simulink model "drone_sim"  (R2021a)
settings: Solver=VariableStepAuto  StartTime=0.0  StopTime=5  MaxStep=0.001  RelTol=1e-7  EnableMultiTasking=on
values from neighbouring files (symbols this model uses):
  arm_length = motorY    (= 0.37)    [drone_6.m]
  batteryDistanceFromCOG = -0.1    [drone_6.m]
  batteryMass = 0.5    [drone_6.m]
  batVolt = 3.7*cells    (= 11.1)    [drone_6.m]
  bodyMass = 0.3    [drone_6.m]
  deadCurrent = 0.3    [drone_6.m]
  h1al = 0.15    [drone_6.m]
  h1iuse = 0    [drone_6.m]
  h1kp = 0    [drone_6.m]
  h1td = 1    [drone_6.m]
  h1ti = 1000    [drone_6.m]
  hoverControl = hoverVoltage/batVolt*1024    [drone_6.m]
  hoverVoltage = hoverCurrent * Ra + hoverRPM / Kv    [drone_6.m]
  hval = 0.2    [drone_6.m]
  hviuse = 0    [drone_6.m]
  hvkp = 50    [drone_6.m]
  hvtd = 1    [drone_6.m]
  hvti = 1    [drone_6.m]
  KDrag = 1.5e-9    (= 1.5e-09)    [drone_6.m]
  Km = 60/(Kv * 2 * pi)    (= 0.013641852265)    [drone_6.m]
  Ktrust = 2.7e-5    (= 2.7e-05)    [drone_6.m]
  minimumMotorVolt = 1.0    (= 1)    [drone_6.m]
  motorMass = 0.102    [drone_6.m]
  N = N + 1    (= 1)    [findp_discrete.m]    (also in findpd_discrete.m = N0; findpi_discrete.m; findpid_discrete.m)
  paal = 0.2    [drone_6.m]
  pakp = 0    [drone_6.m]
  patd = 1    [drone_6.m]
  pati = 100    [drone_6.m]
  pitch_act_lim = 500    [drone_6.m]
  propellerMass = propellerMassRaw + 3*motorInertia/propellerRadius^2    (= 0.019780754243)    [drone_6.m]
  pushOn = 1    [drone_6.m]
  pv_iuse = 0    [drone_6.m]
  pval = 0.4    [drone_6.m]
  pvkp = 0    [drone_6.m]
  pvtd = 1    [drone_6.m]
  pvti = 1    [drone_6.m]
  Ra = 0.083    [drone_6.m]
  raal = 0.25    [drone_6.m]
  rakp = 0    [drone_6.m]
  ral = 0.5    [drone_6.m]
  ratd = 1    [drone_6.m]
  rati = 100    [drone_6.m]
  rkp = 0    [drone_6.m]
  roll_act_lim = 500    [drone_6.m]
  roll_limit = 10    [drone_6.m]
  rtd = 1    [drone_6.m]
  rti = 1    [drone_6.m]
  trust_lim = 1000*0.95    (= 950)    [drone_6.m]
  yaw_act_lim = 500    [drone_6.m]
  yaw_rate_limit = 90    [drone_6.m]
  yawval = 0.3    [drone_6.m]
  yawvkp = 0    [drone_6.m]
  yawvtd = 0    [drone_6.m]
  yawvti = 1    [drone_6.m]
  yawvtiUse = 0    [drone_6.m]
undefined symbols (not defined in the file or in its folder): X, Y, Z
libraries: sm_lib x56, nesl_utility x25, sharedtransform x1
(part 1 of 3)
settings Model: OrderedModelArguments=off  Creator=chr  LastModifiedBy=chr
settings SolverCC: AlgebraicLoopSolver=TrustRegion
settings DataIOCC: LimitDataPoints=on  SaveFormat=Array  ReturnWorkspaceOutputs=off
settings OptimizationCC: LifeSpan=inf
settings DebuggingCC: SFUnexpectedBacktrackingDiag=warning  SFNoUnconditionalDefaultTransitionDiag=warning  SFExecutionAtInitializationDiag=none  SFMachineParentedDataDiag=warning  ArithmeticOperatorsInVariantConditions=warning
settings HardwareCC: ProdBitPerPointer=32  ProdBitPerSizeT=32  ProdBitPerPtrDiffT=32  ProdLargestAtomicFloat=None  ProdIntDivRoundTo=Undefined  ProdEndianess=Unspecified  ProdWordSize=32  ProdHWDeviceType=32-bit Generic
settings ModelReferenceCC: PropagateSignalLabelsOutOfModel=off
settings SFSimCC: SimUseLocalCustomCode=off  CustomCodeUndefinedFunction=UseInterfaceOnly
settings RTWCC: RTWUseLocalCustomCode=off
settings CodeAppCC: StateflowObjectComments=on
settings GRTTargetCC: TargetLangStandard=C89/C90 (ANSI)
settings ConfigComp: CovMetricSettings=dw  CovSaveCumulativeToWorkspaceVar=on  CovSaveSingleToWorkspaceVar=on  CovExternalEMLEnable=off
settings SimscapeCC: SimscapeNormalizeSystem=off  SimscapeLogType=all  SimscapeLogDataHistory=10000
settings ConfigurationSet: Description=SimMechanics 2G
settings ExplorerConfigSet: InternalSimMechanicsExplorerSettings="<ExplorerConfiguration><canonicalview>default</canonicalview><AnimationSetting><BasePlaybackSpeed>1.0</BasePlaybackSpeed><PlaybackSpeedFactor>1.0</PlaybackSpeedFactor></AnimationSetting><TilePanel><TileInfo><Tiles Columns=\"1\" Count=\"1\" Rows=\"1\"><Column Weight=\"1\"/><Row Weight=\"1\"/><Tile Height=\"1\" Width=\"1\" X=\"0\" Y=\"0\"/></Tiles></TileInfo><SceneInfo><SceneViewer><BGColor><R>0.800000011920928955</R><G>0.800000011920928955</G><B>0.800000011920928955</B></BGColor><Camera><DoPerspective>off</DoPerspective><Position><X>-3434.85384488270984</X><Y>-3.87132408808614903</Y><Z>0.619625050913271247</Z></Position><Center><X>-0.134324382199702441</X><Y>-3.87132408808614903</Y><Z>0.619625050913271247</Z></Center><Up><X>0</X><Y>0</Y><Z>1</Z></Up><ViewLimDist>1</ViewLimDist><YLim>2.62838632598170996</YLim><XLim>4.25180140967629594</XLim></Camera></SceneViewer></SceneInfo></TilePanel><MechEditorPanel><Cameras/><GfxPanelCameraMap/><VideoCreator><PlaybackSpeedRatio>1.0</PlaybackSpeedRatio><FrameRate>30</FrameRate><VideoFormat>Motion JPEG AVI</VideoFormat><FrameSize>auto</FrameSize></VideoCreator></MechEditorPanel></ExplorerConfiguration>"

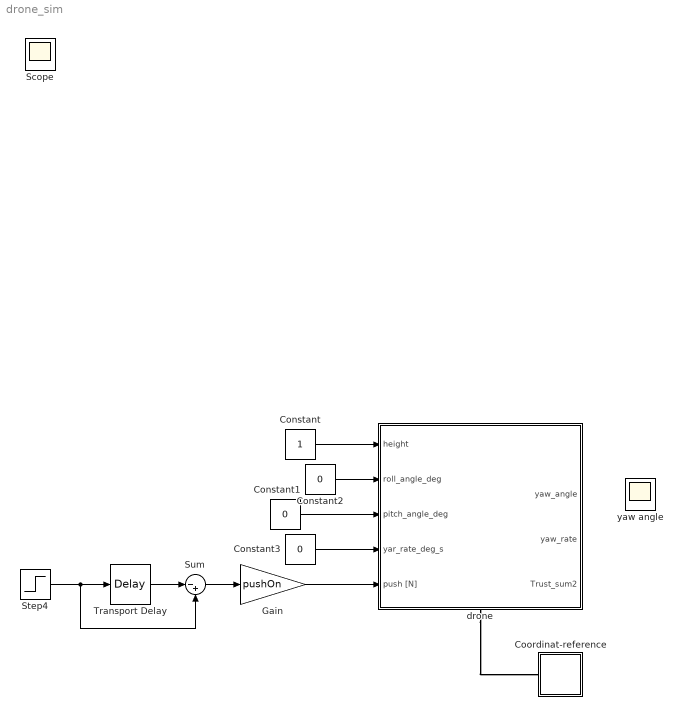
== system drone_sim ==
  Constant : Constant
  Constant1 : Constant  Value=0
  Constant2 : Constant  Value=0
  Constant3 : Constant  Value=0
  Coordinat-reference : Subsystem
  Gain : Gain  Gain=pushOn
  Step4 : Step  Time=2  After=0.2  SampleTime=0
  Sum : Sum  Inputs=|-+
  Transport Delay : TransportDelay  DelayTime=0.2  BufferSize=8196  TransDelayFeedthrough=on
  drone : Subsystem
      settings: PortSchema="{\"entries\":[{\"content\":{\"sides\":[{\"content\":{\"connectorIds\":[\"In1\",\"In2\",\"In3\",\"In4\",\"In5\"]},\"type\":\"ConnectorPlacement.EquallySpacedRectSide\",\"uuid\":\"5594123d-be73-484a-b338-9fd4bc13ca6f\"},{\"content\":{\"connectorIds\":[\"RConn1\",\"Out1\",\"Out2\",\"Out3\"],\"side\":\"RIGHT\"},\"type\":\"ConnectorPlacement.EquallySpacedRectSide\",\"uuid\":\"b12affea-941f-4227-8ac4-f2e96d545e11\"},{\"content\":{\"connectorIds\":[],\"side\":\"TOP\"},\"type\":\"ConnectorPlacement.EquallySpacedRectSide\",\"uuid\":\"44fddaec-2c63-4c5e-8ac9-7d0bb430db34\"},{\"content\":{\"connectorIds\":[\"RConn2\"],\"side\":\"BOTTOM\"},\"type\":\"ConnectorPlacement.EquallySpacedRectSide\",\"uuid\":\"66092044-52c6-48c0-92d2-28ab2c6276b4\"}]},\"type\":\"ConnectorPlacement.EquallySpacedConnector\",\"uuid\":\"500ef50b-769a-4549-99d8-2c1464490163\"}],\"packageUris\":[\"http://schema.mathworks.com/mf0/Connector/R2020b\"],\"version\":\"1.0\"}"
  yaw angle : Scope
  Scope : Scope
  wires:
  Constant/1 -> drone/1(height)
  Step4/1 -> Sum/2, Transport Delay/1
  Transport Delay/1 -> Sum/1
  Sum/1 -> Gain/1
  Constant1/1 -> drone/3(pitch_angle_deg)
  Constant3/1 -> drone/4(yar_rate_deg_s)
  Constant2/1 -> drone/2(roll_angle_deg)
  Gain/1 -> drone/5(push [N])
  connections:
  drone/RConn2 -- Coordinat-reference/RConn1

== system drone_sim/Coordinat-reference ==
  Mechanism Configuration : sm_lib/Utilities/Mechanism Configuration  UniformGravity=Constant  GravityVector=[0 0 -9.82]  GravityVectorUnits=m/s^2  GravityUnits=m/s^2  LinearizationDelta=0.001  JointModeTransitionNonlinearIterations=2
  Solver Configuration : nesl_utility/Solver Configuration  PhysicalDomain=network_engine_domain  SubClassName=solver  LeftPortType=input  RightPortType=generic  Tones=[]  Harmonics=[]  SimulateNoise=off  Profile=off  UseLocalSampling=off  EnableSwitchedLinearOptims=on  FrequencyDomain=off  UseCCode=off  RelTol=0.001  AbsTol=1e-06  MinStep=1e-09  ToWorkspace=off  RevertToSquareIcSolve=off  NumHomotopyIterations=100  PhasorMode=off  PhasorModeNumHarmonics=1  DoDC=off  ResidualTolerance=1e-09  UseLocalSolver=off  LocalSolverChoice=NE_BACKWARD_EULER_ADVANCER  LocalSolverSampleTime=0.001  DoFixedCost=off  MaxNonlinIter=3  MaxModeIter=2  ComputeImpulses=off  ImpulseIterations=2  LinearAlgebra=Sparse  EquationFormulation=NE_TIME_EF  DelaysMemoryBudget=1024  AutomaticFiltering=on  FilteringTimeConstant=0.001  PartitionStorageMethod=AS_NEEDED  PartitionMemoryBudget=1024  PartitionMethod=FAST
      settings: SourceProductBaseCode=PW,SS
  World Frame : sm_lib/Frames and Transforms/World Frame
  ground : sm_lib/Body Elements/Brick Solid  GraphicAmbientColor=[0.15 0.15 0.15 1.0]  BasedOnType=Mass  BrickDimensions=[1 1 0.01]  BrickDimensionUnits=m  CenterOfMass=[0 0 0]  CenterOfMassUnits=m  GraphicDiffuseColor=[0.2 0.5 0.2]  Density=1000  DensityUnits=kg/(m^3)  DoExposeReferenceFrame=on  GraphicEmissiveColor=[0.0 0.0 0.0 1.0]  ExportEntireGeometry=off  SerializedFrames=<Frames/>  MarkerShape=Sphere  MarkerSize=10  GraphicType=FromGeometry  InertiaType=CalculateFromGeometry  Mass=1  MassUnits=kg  MomentsOfInertia=[1 1 1]  MomentsOfInertiaUnits=kg*m^2  GraphicOpacity=1.0  ProductsOfInertia=[0 0 0]  ProductsOfInertiaUnits=kg*m^2  GraphicShininess=75  GraphicSpecularColor=[0.5 0.5 0.5 1.0]  GraphicVisPropType=SimpleVisualProperties
  GND : PMIOPort  Side=Right
  connections:
  Solver Configuration/RConn1 -- GND/RConn1 -- ground/RConn1 -- World Frame/RConn1 -- Mechanism Configuration/RConn1

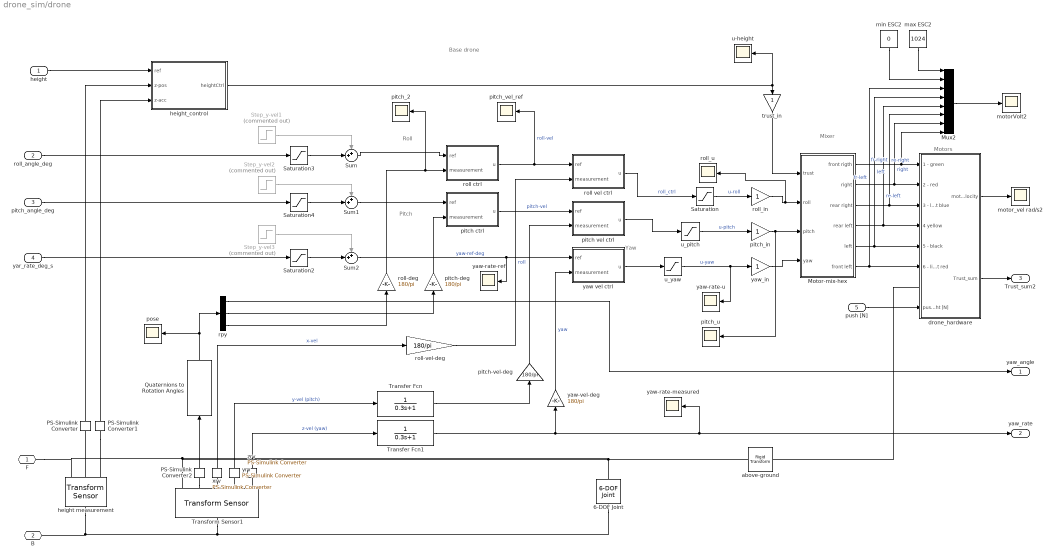
== system drone_sim/drone ==
  note: Base drone
  note: Yaw
  note: Pitch
  note: Roll
  note: Motors
  note: Mixer
  height : Inport
  roll_angle_deg : Inport  Port=2
  pitch_angle_deg : Inport  Port=3
  yar_rate_deg_s : Inport  Port=4
  push [N] : Inport  Port=5
  6-DOF Joint : sm_lib/Joints/6-DOF Joint  JointMode=Normal  SenseConstraintForce=off  SenseConstraintForceX=off  SenseConstraintForceY=off  SenseConstraintForceZ=off  SenseConstraintTorque=off  SenseConstraintTorqueX=off  SenseConstraintTorqueY=off  SenseConstraintTorqueZ=off  SenseTotalForce=off  SenseTotalForceX=off  SenseTotalForceY=off  SenseTotalForceZ=off  SenseTotalTorque=off  SenseTotalTorqueX=off  SenseTotalTorqueY=off  SenseTotalTorqueZ=off  CompositeWrenchDir=FollowerOnBase  CompositeWrenchFrame=BaseFrame  PxEquilibriumPosition=0  PxEquilibriumPositionUnits=m  PxSpringStiffness=0  PxSpringStiffnessUnits=N/m  PxDampingCoefficient=0  PxDampingCoefficientUnits=N/(m/s)  PxTorqueActuationMode=NoTorque  PxMotionActuationMode=ComputedMotion  PxSensePosition=off  PxSenseVelocity=off  PxSenseAcceleration=off  PxSenseTorqueForce=off  PxSenseLowerLimitTorqueForce=off  PxSenseUpperLimitTorqueForce=off  PxLowerLimitSpecify=off  PxLowerLimitBound=-1  PxLowerLimitBoundUnits=m  PxLowerLimitStiffness=1e6  PxLowerLimitStiffnessUnits=N/m  PxLowerLimitDamping=1e3  PxLowerLimitDampingUnits=N/(m/s)  PxLowerLimitTransitionRegionWidth=1e-4  PxLowerLimitTransitionRegionWidthUnits=m  PxUpperLimitSpecify=off  PxUpperLimitBound=1  PxUpperLimitBoundUnits=m  PxUpperLimitStiffness=1e6  PxUpperLimitStiffnessUnits=N/m  PxUpperLimitDamping=1e3  PxUpperLimitDampingUnits=N/(m/s)  PxUpperLimitTransitionRegionWidth=1e-4  PxUpperLimitTransitionRegionWidthUnits=m  PxPositionTargetSpecify=off  PxPositionTargetPriority=High  PxPositionTargetValue=0  PxPositionTargetValueUnits=m  PxVelocityTargetSpecify=off  PxVelocityTargetPriority=High  PxVelocityTargetValue=0  PxVelocityTargetValueUnits=m/s  PyEquilibriumPosition=0  PyEquilibriumPositionUnits=m  PySpringStiffness=0  PySpringStiffnessUnits=N/m  PyDampingCoefficient=0  PyDampingCoefficientUnits=N/(m/s)  PyTorqueActuationMode=NoTorque  PyMotionActuationMode=ComputedMotion  PySensePosition=off  PySenseVelocity=off  PySenseAcceleration=off  PySenseTorqueForce=off  PySenseLowerLimitTorqueForce=off  PySenseUpperLimitTorqueForce=off  PyLowerLimitSpecify=off  PyLowerLimitBound=-1  PyLowerLimitBoundUnits=m  PyLowerLimitStiffness=1e6  PyLowerLimitStiffnessUnits=N/m  PyLowerLimitDamping=1e3  PyLowerLimitDampingUnits=N/(m/s)  PyLowerLimitTransitionRegionWidth=1e-4  PyLowerLimitTransitionRegionWidthUnits=m  PyUpperLimitSpecify=off  PyUpperLimitBound=1  PyUpperLimitBoundUnits=m  PyUpperLimitStiffness=1e6  PyUpperLimitStiffnessUnits=N/m  PyUpperLimitDamping=1e3  PyUpperLimitDampingUnits=N/(m/s)  PyUpperLimitTransitionRegionWidth=1e-4  PyUpperLimitTransitionRegionWidthUnits=m  PyPositionTargetSpecify=off  PyPositionTargetPriority=High  PyPositionTargetValue=0  PyPositionTargetValueUnits=m  PyVelocityTargetSpecify=off  PyVelocityTargetPriority=High  PyVelocityTargetValue=0  PyVelocityTargetValueUnits=m/s  PzEquilibriumPosition=0  PzEquilibriumPositionUnits=m  PzSpringStiffness=0  PzSpringStiffnessUnits=N/m  PzDampingCoefficient=0  PzDampingCoefficientUnits=N/(m/s)  PzTorqueActuationMode=NoTorque  PzMotionActuationMode=ComputedMotion  PzSensePosition=off  PzSenseVelocity=off  PzSenseAcceleration=off  PzSenseTorqueForce=off  PzSenseLowerLimitTorqueForce=off  PzSenseUpperLimitTorqueForce=off  PzLowerLimitSpecify=off  PzLowerLimitBound=-1  PzLowerLimitBoundUnits=m  PzLowerLimitStiffness=1e6  PzLowerLimitStiffnessUnits=N/m  PzLowerLimitDamping=1e3  PzLowerLimitDampingUnits=N/(m/s)  PzLowerLimitTransitionRegionWidth=1e-4  PzLowerLimitTransitionRegionWidthUnits=m  PzUpperLimitSpecify=off  PzUpperLimitBound=1  PzUpperLimitBoundUnits=m  PzUpperLimitStiffness=1e6  PzUpperLimitStiffnessUnits=N/m  PzUpperLimitDamping=1e3  PzUpperLimitDampingUnits=N/(m/s)  PzUpperLimitTransitionRegionWidth=1e-4  PzUpperLimitTransitionRegionWidthUnits=m  PzPositionTargetSpecify=off  PzPositionTargetPriority=High  PzPositionTargetValue=0  PzPositionTargetValueUnits=m  PzVelocityTargetSpecify=off  PzVelocityTargetPriority=High  PzVelocityTargetValue=0  PzVelocityTargetValueUnits=m/s  SphDefPosRotationMethod=None  SphDefPosRotationAngleUnits=deg  SphDefPosRotationStandardAxis=+Z  SphDefPosRotationAngle=0.0  SphDefPosRotationArbitraryAxis=[0 0 1]  SphDefPosFollAlignAxisA=+X  SphDefPosBaseAlignAxisA=+Y  SphDefPosFollAlignAxisB=+Y  SphDefPosBaseAlignAxisB=+Z  SphDefPosRotationSequenceAxes=FollowerAxes  SphDefPosRotationSequence=XYX  SphDefPosRotationSequenceAngles=[0 0 0]  SphDefPosRotationSequenceAnglesUnits=deg  SphDefPosRotationMatrix=[1 0 0; 0 1 0; 0 0 1]  SphEqPosRotationMethod=None  SphEqPosRotationAngleUnits=deg  SphEqPosRotationStandardAxis=+Z  SphEqPosRotationAngle=0.0  SphEqPosRotationArbitraryAxis=[0 0 1]  SphEqPosFollAlignAxisA=+X  SphEqPosBaseAlignAxisA=+Y  SphEqPosFollAlignAxisB=+Y  SphEqPosBaseAlignAxisB=+Z  SphEqPosRotationSequenceAxes=FollowerAxes  SphEqPosRotationSequence=XYX  SphEqPosRotationSequenceAngles=[0 0 0]  SphEqPosRotationSequenceAnglesUnits=deg  SphEqPosRotationMatrix=[1 0 0; 0 1 0; 0 0 1]  SphSpringStiffness=0  SphSpringStiffnessUnits=N*m/deg  SphDampingCoefficient=0  SphDampingCoefficientUnits=N*m/(deg/s)  SphActuateTorqueX=off  SphActuateTorqueY=off  SphActuateTorqueZ=off  SphActuateTorque=off  SphTorqueActuationMode=NoTorque  SphMotionActuationMode=ComputedMotion  SphActuationFrame=BaseFrame  SphSensePosition=off  SphSenseVelocityX=off  SphSenseVelocityY=off  SphSenseVelocityZ=off  SphSenseVelocity=off  SphSenseAccelerationX=off  SphSenseAccelerationY=off  SphSenseAccelerationZ=off  SphSenseAcceleration=off  SphSenseTorqueX=off  SphSenseTorqueY=off  SphSenseTorqueZ=off  SphSenseTorqueForce=off  SphSenseLowerLimitTorqueMag=off  SphSenseUpperLimitTorqueMag=off  SphSensingFrame=BaseFrame  SphLowerLimitSpecify=off  SphLowerLimitBound=15  SphLowerLimitBoundUnits=deg  SphLowerLimitStiffness=1e4  SphLowerLimitStiffnessUnits=N*m/deg  SphLowerLimitDamping=10  SphLowerLimitDampingUnits=N*m/(deg/s)  SphLowerLimitTransitionRegionWidth=0.1  SphLowerLimitTransitionRegionWidthUnits=deg  SphUpperLimitSpecify=off  SphUpperLimitBound=45  SphUpperLimitBoundUnits=deg  SphUpperLimitStiffness=1e4  SphUpperLimitStiffnessUnits=N*m/deg  SphUpperLimitDamping=10  SphUpperLimitDampingUnits=N*m/(deg/s)  SphUpperLimitTransitionRegionWidth=0.1  SphUpperLimitTransitionRegionWidthUnits=deg  SphPositionTargetRotationMethod=None  SphPositionTargetRotationAngleUnits=deg  SphPositionTargetRotationStandardAxis=+Z  SphPositionTargetRotationAngle=0.0  SphPositionTargetRotationArbitraryAxis=[0 0 1]  SphPositionTargetFollAlignAxisA=+X  SphPositionTargetBaseAlignAxisA=+Y  SphPositionTargetFollAlignAxisB=+Y  SphPositionTargetBaseAlignAxisB=+Z  SphPositionTargetRotationSequenceAxes=FollowerAxes  SphPositionTargetRotationSequence=XYX  SphPositionTargetRotationSequenceAngles=[0 0 0]  SphPositionTargetRotationSequenceAnglesUnits=deg  SphPositionTargetRotationMatrix=[1 0 0; 0 1 0; 0 0 1]  SphPositionTargetSpecify=off  SphPositionTargetPriority=High  SphVelocityTargetValue=[0 0 0]  SphVelocityTargetValueUnits=deg/s  SphVelocityTargetSpecify=off  SphVelocityTargetPriority=High  SphVelocityTargetInFollowerFrame=on
  Motor-mix-hex : Subsystem
  Mux2 : Mux  Inputs=8
  PS-Simulink Converter : nesl_utility/PS-Simulink Converter  PhysicalDomain=network_engine_domain  SubClassName=ps_output  LeftPortType=input  RightPortType=output  PseudoPeriodic=off  Frequencies=[]  Unit=inherit  AffineConversion=off
      settings: SourceProductBaseCode=PW,SS
  PS-Simulink Converter1 : nesl_utility/PS-Simulink Converter  PhysicalDomain=network_engine_domain  SubClassName=ps_output  LeftPortType=input  RightPortType=output  PseudoPeriodic=off  Frequencies=[]  Unit=inherit  AffineConversion=off
      settings: SourceProductBaseCode=PW,SS
  PS-Simulink Converter2 : nesl_utility/PS-Simulink Converter  PhysicalDomain=network_engine_domain  SubClassName=ps_output  LeftPortType=input  RightPortType=output  PseudoPeriodic=off  Frequencies=[]  Unit=inherit  AffineConversion=off
      settings: SourceProductBaseCode=PW,SS
  Quaternions to Rotation Angles : sharedtransform/Quaternions to Rotation Angles  rotationOrder=ZYX  aMode=aMode
      settings: SourceProductBaseCode=AE,PW,DR,MT,UV,VE
  Saturation : Saturate  UpperLimit=roll_act_lim  LowerLimit=-roll_act_lim
  Saturation2 : Saturate  UpperLimit=yaw_rate_limit  LowerLimit=-yaw_rate_limit
  Saturation3 : Saturate  UpperLimit=roll_limit  LowerLimit=-roll_limit
  Saturation4 : Saturate  UpperLimit=roll_limit  LowerLimit=-roll_limit
  Step_y-vel1 : Step  Commented=on  Time=3  After=2  SampleTime=0
  Step_y-vel2 : Step  Commented=on  Time=3  After=0.5  SampleTime=0
  Step_y-vel3 : Step  Commented=on  Time=3  After=15  SampleTime=0
  Sum : Sum  Inputs=++|
  Sum1 : Sum  Inputs=++|
  Sum2 : Sum  Inputs=++|
  Transfer Fcn : TransferFcn  Denominator=[0.3 1]
  Transfer Fcn1 : TransferFcn  Denominator=[0.3 1]
  Transform Sensor1 : sm_lib/Frames and Transforms/Transform Sensor  MeasurementFrame=Follower  SenseAngle=off  SenseAxis=off  SenseAngle1=off  SenseAngle2=off  SenseAngle3=off  SenseQ=on  SenseR=off  SenseOmegaX=on  SenseOmegaY=on  SenseOmegaZ=on  SenseOmega1=off  SenseOmega2=off  SenseOmega3=off  SenseQDot=off  SenseRDot=off  SenseAlphaX=off  SenseAlphaY=off  SenseAlphaZ=off  SenseAlpha1=off  SenseAlpha2=off  SenseAlpha3=off  SenseQDDot=off  SenseRDDot=off  SenseX=off  SenseY=off  SenseZ=off  SenseRad=off  SenseAzim=off  SenseDist=off  SenseInc=off  SenseXDot=off  SenseYDot=off  SenseZDot=off  SenseRadDot=off  SenseAzimDot=off  SenseDistDot=off  SenseIncDot=off  SenseXDDot=off  SenseYDDot=off  SenseZDDot=off  SenseRadDDot=off  SenseAzimDDot=off  SenseDistDDot=off  SenseIncDDot=off
  above-ground : sm_lib/Frames and Transforms/Rigid Transform  TranslationMethod=StandardAxis  TranslationStandardOffset=0.02  TranslationLengthUnit=m  TranslationStandardAxis=+Z  TranslationCartesianOffset=[0.14 0.14 0.03]  TranslationROffset=arm_length  TranslationROffsetUnits=m  TranslationZOffset=0.03  TranslationZOffsetUnits=m  TranslationThetaOffset=-150  TranslationThetaOffsetUnits=deg  RotationMethod=None  RotationAngleUnits=deg  RotationStandardAxis=+Z  RotationAngle=0.05  RotationArbitraryAxis=[0 0 1]  FollAlignAxisA=+X  BaseAlignAxisA=+Y  FollAlignAxisB=+Y  BaseAlignAxisB=+Z  RotationSequenceAxes=FollowerAxes  RotationSequence=XYX  RotationSequenceAngles=[0 0 0]  RotationSequenceAnglesUnits=deg  RotationMatrix=[1 0 0; 0 1 0; 0 0 1]
  drone_hardware : Subsystem
      settings: PortSchema="{\"entries\":[{\"content\":{\"sides\":[{\"content\":{\"connectorIds\":[\"In1\",\"In2\",\"In3\",\"In4\",\"In5\",\"In6\",\"LConn1\",\"In7\"]},\"type\":\"ConnectorPlacement.EquallySpacedRectSide\",\"uuid\":\"51e20491-184f-4c13-ad67-858d0ecfecfd\"},{\"content\":{\"connectorIds\":[\"Out1\",\"Out2\"],\"side\":\"RIGHT\"},\"type\":\"ConnectorPlacement.EquallySpacedRectSide\",\"uuid\":\"dd38fec1-9b5b-4065-9c26-bdf68d278980\"},{\"content\":{\"connectorIds\":[],\"side\":\"TOP\"},\"type\":\"ConnectorPlacement.EquallySpacedRectSide\",\"uuid\":\"f644b8cb-3aa9-4068-acaf-6a442e3f1948\"}]},\"type\":\"ConnectorPlacement.EquallySpacedConnector\",\"uuid\":\"e398b018-d970-47a6-aa8b-d81f44328f20\"}],\"packageUris\":[\"http://schema.mathworks.com/mf0/Connector/19700101\"],\"version\":\"1.0\"}"
  height measurement : sm_lib/Frames and Transforms/Transform Sensor  MeasurementFrame=World  SenseAngle=off  SenseAxis=off  SenseAngle1=off  SenseAngle2=off  SenseAngle3=off  SenseQ=off  SenseR=off  SenseOmegaX=off  SenseOmegaY=off  SenseOmegaZ=off  SenseOmega1=off  SenseOmega2=off  SenseOmega3=off  SenseQDot=off  SenseRDot=off  SenseAlphaX=off  SenseAlphaY=off  SenseAlphaZ=off  SenseAlpha1=off  SenseAlpha2=off  SenseAlpha3=off  SenseQDDot=off  SenseRDDot=off  SenseX=off  SenseY=off  SenseZ=on  SenseRad=off  SenseAzim=off  SenseDist=off  SenseInc=off  SenseXDot=off  SenseYDot=off  SenseZDot=off  SenseRadDot=off  SenseAzimDot=off  SenseDistDot=off  SenseIncDot=off  SenseXDDot=off  SenseYDDot=off  SenseZDDot=on  SenseRadDDot=off  SenseAzimDDot=off  SenseDistDDot=off  SenseIncDDot=off
  height_control : Subsystem
  max ESC2 : Constant  Value=1024
  min ESC2 : Constant  Value=0
  motorVolt2 : Scope
  motor_vel rad/s2 : Scope
  pitch ctrl : Subsystem
  pitch vel ctrl : Subsystem
  pitch-deg : Gain  Gain=180/pi
  pitch-vel-deg : Gain  Gain=180/pi
  pitch_2 : Scope
  pitch_in : Gain
  pitch_u : Scope
  pitch_vel_ref : Scope
  pose : Scope
  roll ctrl : Subsystem
  roll vel ctrl : Subsystem
  roll-deg : Gain  Gain=180/pi
  roll-vel-deg : Gain  Gain=180/pi
  roll_in : Gain
  roll_u : Scope
  rpy : Demux  Outputs=3
  trust_in : Gain
  u-height : Scope
  u_pitch : Saturate  UpperLimit=pitch_act_lim  LowerLimit=-pitch_act_lim
  u_yaw : Saturate  UpperLimit=yaw_act_lim  LowerLimit=-yaw_act_lim
  xrv : nesl_utility/PS-Simulink Converter  PhysicalDomain=network_engine_domain  SubClassName=ps_output  LeftPortType=input  RightPortType=output  PseudoPeriodic=off  Frequencies=[]  Unit=inherit  AffineConversion=off
      settings: SourceProductBaseCode=PW,SS
  yaw vel ctrl : Subsystem
  yaw-rate-measured : Scope
  yaw-rate-ref : Scope
  yaw-rate-u : Scope
  yaw-vel-deg : Gain  Gain=180/pi
  yaw_in : Gain
  yrv : nesl_utility/PS-Simulink Converter  PhysicalDomain=network_engine_domain  SubClassName=ps_output  LeftPortType=input  RightPortType=output  PseudoPeriodic=off  Frequencies=[]  Unit=inherit  AffineConversion=off
      settings: SourceProductBaseCode=PW,SS
  zrv : nesl_utility/PS-Simulink Converter  PhysicalDomain=network_engine_domain  SubClassName=ps_output  LeftPortType=input  RightPortType=output  PseudoPeriodic=off  Frequencies=[]  Unit=inherit  AffineConversion=off
      settings: SourceProductBaseCode=PW,SS
  F : PMIOPort  Side=Right
  B : PMIOPort  Port=2  Side=Right
  yaw_angle : Outport
  yaw_rate : Outport  Port=2
  Trust_sum2 : Outport  Port=3
  wires:
  Sum1/1 -> pitch ctrl/1(ref)
  rpy/2 -> pitch-deg/1
  rpy/3 -> roll-deg/1
  trust_in/1 -> Motor-mix-hex/1(trust)
  yrv/1 -> Transfer Fcn/1  "y-vel (pitch)"
  pitch_in/1 -> pitch_u/1, Motor-mix-hex/3(pitch)
  Saturation4/1 -> Sum1/2
  Sum/1 -> roll ctrl/1(ref)
  PS-Simulink Converter1/1 -> height_control/3(z-acc)
  yaw-vel-deg/1 -> yaw vel ctrl/2(measurement)  "yaw"
  xrv/1 -> roll-vel-deg/1  "x-vel"
  Step_y-vel2/1 -> Sum1/1
  Saturation3/1 -> Sum/2
  roll ctrl/1(u) -> pitch_vel_ref/1, roll vel ctrl/1(ref)  "roll-vel"
  pitch-vel-deg/1 -> pitch vel ctrl/2(measurement)
  pitch vel ctrl/1(u) -> u_pitch/1
  yar_rate_deg_s/1 -> Saturation2/1
  Step_y-vel3/1 -> Sum2/1
  zrv/1 -> Transfer Fcn1/1  "z-vel (yaw)"
  PS-Simulink Converter2/1 -> Quaternions to Rotation Angles/1
  Transfer Fcn/1 -> pitch-vel-deg/1
  u_yaw/1 -> yaw-rate-u/1, yaw_in/1  "u-yaw"
  Saturation/1 -> roll_in/1  "u-roll"
  yaw vel ctrl/1(u) -> u_yaw/1
  height/1 -> height_control/1(ref)
  roll_in/1 -> roll_u/1, Motor-mix-hex/2(roll)
  pitch ctrl/1(u) -> pitch vel ctrl/1(ref)  "pitch-vel"
  Saturation2/1 -> Sum2/2
  roll_angle_deg/1 -> Saturation3/1
  Transfer Fcn1/1 -> yaw-vel-deg/1, yaw-rate-measured/1, yaw_rate/1
  pitch-deg/1 -> pitch ctrl/2(measurement)
  height_control/1(heightCtrl) -> u-height/1, trust_in/1
  Quaternions to Rotation Angles/1 -> pose/1, rpy/1
  pitch_angle_deg/1 -> Saturation4/1
  u_pitch/1 -> pitch_in/1  "u-pitch"
  Step_y-vel1/1 -> Sum/1
  Sum2/1 -> yaw-rate-ref/1, yaw vel ctrl/1(ref)  "yaw-ref-deg"
  roll-deg/1 -> pitch_2/1, roll ctrl/2(measurement)
  yaw_in/1 -> Motor-mix-hex/4(yaw)
  PS-Simulink Converter/1 -> height_control/2(z-pos)
  roll vel ctrl/1(u) -> Saturation/1  "roll_ctrl"
  roll-vel-deg/1 -> roll vel ctrl/2(measurement)  "roll"
  rpy/1 -> yaw_angle/1
  push [N]/1 -> drone_hardware/7(push right [N])
  max ESC2/1 -> Mux2/1
  Motor-mix-hex/5(left) -> Mux2/4, drone_hardware/5(5 - black)  "left"
  Motor-mix-hex/6(front left) -> Mux2/3, drone_hardware/6(6 - light red)  "fr-left"
  drone_hardware/1(motor_velocity) -> motor_vel rad/s2/1
  Motor-mix-hex/1(front rigth) -> Mux2/8, drone_hardware/1(1 - green)  "fr-right"
  Motor-mix-hex/3(rear right) -> Mux2/6, drone_hardware/3(3 - light blue)  "re-right"
  drone_hardware/2(Trust_sum) -> Trust_sum2/1
  Mux2/1 -> motorVolt2/1
  Motor-mix-hex/4(rear left) -> Mux2/5, drone_hardware/4(4 yellow)  "re-left"
  min ESC2/1 -> Mux2/2
  Motor-mix-hex/2(right) -> Mux2/7, drone_hardware/2(2 - red)  "right"
  connections:
  PS-Simulink Converter2/LConn1 -- Transform Sensor1/RConn2
  drone_hardware/LConn1 -- above-ground/RConn1
  zrv/LConn1 -- Transform Sensor1/RConn5
  6-DOF Joint/RConn1 -- F/RConn1 -- height measurement/RConn1 -- Transform Sensor1/RConn1 -- above-ground/LConn1
  6-DOF Joint/LConn1 -- Transform Sensor1/LConn1 -- height measurement/LConn1 -- B/RConn1
  PS-Simulink Converter1/LConn1 -- height measurement/RConn3
  yrv/LConn1 -- Transform Sensor1/RConn4
  xrv/LConn1 -- Transform Sensor1/RConn3
  height measurement/RConn2 -- PS-Simulink Converter/LConn1

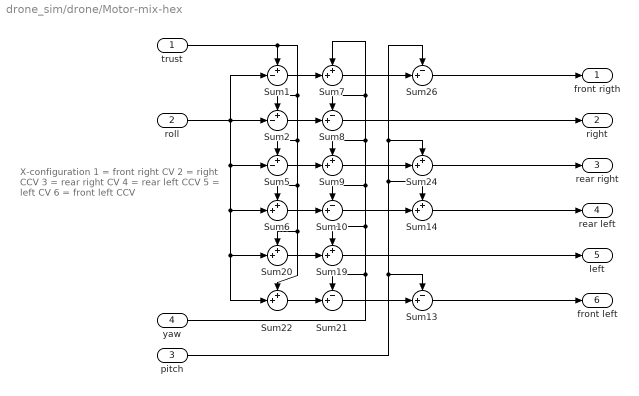
== system drone_sim/drone/Motor-mix-hex ==
  note: X-configuration
      | 1 = front right CV
      | 2 = right        CCV
      | 3 = rear right CV
      | 4 = rear left   CCV
      | 5 = left          CV
      | 6 = front left CCV
  trust : Inport
  roll : Inport  Port=2
  pitch : Inport  Port=3
  yaw : Inport  Port=4
  Sum1 : Sum  Inputs=+-|
  Sum{8,10,13,21,26} (5 alike) : Sum  Inputs=-+|
  Sum{6..7,9,14,19..20,22,24} (8 alike) : Sum  Inputs=++|
  Sum2 : Sum  Inputs=+-|
  Sum5 : Sum  Inputs=+-|
  front rigth : Outport
  right : Outport  Port=2
  rear right : Outport  Port=3
  rear left : Outport  Port=4
  left : Outport  Port=5
  front left : Outport  Port=6
  wires:
  trust/1 -> Sum22/1, Sum20/1, Sum6/1, Sum5/1, Sum2/1, Sum1/1
  Sum2/1 -> Sum8/2
  Sum22/1 -> Sum21/2
  Sum1/1 -> Sum7/2
  yaw/1 -> Sum21/1, Sum7/1, Sum8/1, Sum9/1, Sum10/1, Sum19/1
  Sum5/1 -> Sum9/2
  Sum21/1 -> Sum13/2
  Sum6/1 -> Sum10/2
  Sum7/1 -> Sum26/2
  Sum9/1 -> Sum24/2
  Sum20/1 -> Sum19/2
  Sum10/1 -> Sum14/2
  roll/1 -> Sum22/2, Sum20/2, Sum6/2, Sum5/2, Sum1/2, Sum2/2
  pitch/1 -> Sum14/1, Sum24/1, Sum26/1, Sum13/1
  Sum13/1 -> front left/1
  Sum19/1 -> left/1
  Sum14/1 -> rear left/1
  Sum24/1 -> rear right/1
  Sum8/1 -> right/1
  Sum26/1 -> front rigth/1

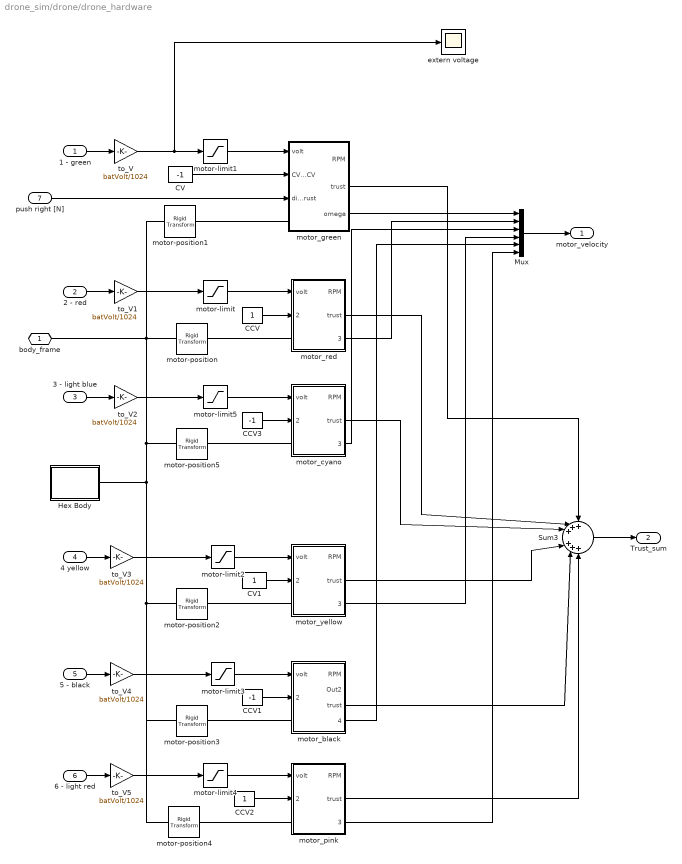
== system drone_sim/drone/drone_hardware ==
  1 - green : Inport
  2 - red : Inport  Port=2
  3 - light blue : Inport  Port=3
  4 yellow : Inport  Port=4
  5 - black : Inport  Port=5
  6 - light red : Inport  Port=6
  push right [N] : Inport  Port=7
  CCV : Constant
  CCV1 : Constant  Value=-1
  CCV2 : Constant
  CCV3 : Constant  Value=-1
  CV : Constant  Value=-1
  CV1 : Constant
  Hex Body : Subsystem
      settings: PortSchema="{\"entries\":[{\"content\":{\"sides\":[{\"content\":{\"connectorIds\":[]},\"type\":\"ConnectorPlacement.EquallySpacedRectSide\",\"uuid\":\"01ed8a62-6d0e-429c-9fb0-ca702bbee18e\"},{\"content\":{\"connectorIds\":[],\"side\":\"RIGHT\"},\"type\":\"ConnectorPlacement.EquallySpacedRectSide\",\"uuid\":\"cdf1885d-1c5d-45e3-9572-3c603101c78e\"},{\"content\":{\"connectorIds\":[],\"side\":\"TOP\"},\"type\":\"ConnectorPlacement.EquallySpacedRectSide\",\"uuid\":\"9e81d776-774a-44d3-a154-58f7c6a5d82e\"},{\"content\":{\"connectorIds\":[\"RConn1\"],\"side\":\"BOTTOM\"},\"type\":\"ConnectorPlacement.EquallySpacedRectSide\",\"uuid\":\"9aef484f-1b98-4f15-b054-c09d0dce9b9e\"}]},\"type\":\"ConnectorPlacement.EquallySpacedConnector\",\"uuid\":\"2bac5469-8928-4e08-b1cb-20bc7858b0f9\"}],\"packageUris\":[\"http://schema.mathworks.com/mf0/Connector/19700101\"],\"version\":\"1.0\"}"
  Mux : Mux  Inputs=6
  Sum3 : Sum  Inputs=+++|+++
  extern voltage : Scope
  motor-limit{,1..5} (6 alike) : Saturate  UpperLimit=batVolt  LowerLimit=minimumMotorVolt
  motor-position : sm_lib/Frames and Transforms/Rigid Transform  TranslationMethod=Cylindrical  TranslationStandardOffset=0  TranslationLengthUnit=m  TranslationStandardAxis=+Z  TranslationCartesianOffset=[0 0.2 0.03]  TranslationROffset=arm_length  TranslationROffsetUnits=m  TranslationZOffset=0.03  TranslationZOffsetUnits=m  TranslationThetaOffset=-90  TranslationThetaOffsetUnits=deg  RotationMethod=StandardAxis  RotationAngleUnits=deg  RotationStandardAxis=+Y  RotationAngle=0.0  RotationArbitraryAxis=[0 0 1]  FollAlignAxisA=+X  BaseAlignAxisA=+Y  FollAlignAxisB=+Y  BaseAlignAxisB=+Z  RotationSequenceAxes=FollowerAxes  RotationSequence=XYX  RotationSequenceAngles=[0 0 0]  RotationSequenceAnglesUnits=deg  RotationMatrix=[1 0 0; 0 1 0; 0 0 1]
  motor-position1 : sm_lib/Frames and Transforms/Rigid Transform  TranslationMethod=Cylindrical  TranslationStandardOffset=0  TranslationLengthUnit=m  TranslationStandardAxis=+Z  TranslationCartesianOffset=[0 -0.2 0.03]  TranslationROffset=arm_length  TranslationROffsetUnits=m  TranslationZOffset=0.03  TranslationZOffsetUnits=m  TranslationThetaOffset=-30  TranslationThetaOffsetUnits=deg  RotationMethod=StandardAxis  RotationAngleUnits=deg  RotationStandardAxis=+Y  RotationAngle=0.0  RotationArbitraryAxis=[0 0 1]  FollAlignAxisA=+X  BaseAlignAxisA=+Y  FollAlignAxisB=+Y  BaseAlignAxisB=+Z  RotationSequenceAxes=FollowerAxes  RotationSequence=XYX  RotationSequenceAngles=[0 0 0]  RotationSequenceAnglesUnits=deg  RotationMatrix=[1 0 0; 0 1 0; 0 0 1]
  motor-position2 : sm_lib/Frames and Transforms/Rigid Transform  TranslationMethod=Cylindrical  TranslationStandardOffset=0  TranslationLengthUnit=m  TranslationStandardAxis=+Z  TranslationCartesianOffset=[0.2 0. 0.03]  TranslationROffset=arm_length  TranslationROffsetUnits=m  TranslationZOffset=0.03  TranslationZOffsetUnits=m  TranslationThetaOffset=+150  TranslationThetaOffsetUnits=deg  RotationMethod=StandardAxis  RotationAngleUnits=deg  RotationStandardAxis=+Y  RotationAngle=0.0  RotationArbitraryAxis=[0 0 1]  FollAlignAxisA=+X  BaseAlignAxisA=+Y  FollAlignAxisB=+Y  BaseAlignAxisB=+Z  RotationSequenceAxes=FollowerAxes  RotationSequence=XYX  RotationSequenceAngles=[0 0 0]  RotationSequenceAnglesUnits=deg  RotationMatrix=[1 0 0; 0 1 0; 0 0 1]
  motor-position3 : sm_lib/Frames and Transforms/Rigid Transform  TranslationMethod=Cylindrical  TranslationStandardOffset=0  TranslationLengthUnit=m  TranslationStandardAxis=+Z  TranslationCartesianOffset=[-0.2 0. 0.03]  TranslationROffset=arm_length  TranslationROffsetUnits=m  TranslationZOffset=0.03  TranslationZOffsetUnits=m  TranslationThetaOffset=90  TranslationThetaOffsetUnits=deg  RotationMethod=StandardAxis  RotationAngleUnits=deg  RotationStandardAxis=+Y  RotationAngle=0.0  RotationArbitraryAxis=[0 0 1]  FollAlignAxisA=+X  BaseAlignAxisA=+Y  FollAlignAxisB=+Y  BaseAlignAxisB=+Z  RotationSequenceAxes=FollowerAxes  RotationSequence=XYX  RotationSequenceAngles=[0 0 0]  RotationSequenceAnglesUnits=deg  RotationMatrix=[1 0 0; 0 1 0; 0 0 1]
  motor-position4 : sm_lib/Frames and Transforms/Rigid Transform  TranslationMethod=Cylindrical  TranslationStandardOffset=0  TranslationLengthUnit=m  TranslationStandardAxis=+Z  TranslationCartesianOffset=[-0.14 -0.14 0.03]  TranslationROffset=arm_length  TranslationROffsetUnits=m  TranslationZOffset=0.03  TranslationZOffsetUnits=m  TranslationThetaOffset=30  TranslationThetaOffsetUnits=deg  RotationMethod=StandardAxis  RotationAngleUnits=deg  RotationStandardAxis=+Y  RotationAngle=0.0  RotationArbitraryAxis=[0 0 1]  FollAlignAxisA=+X  BaseAlignAxisA=+Y  FollAlignAxisB=+Y  BaseAlignAxisB=+Z  RotationSequenceAxes=FollowerAxes  RotationSequence=XYX  RotationSequenceAngles=[0 0 0]  RotationSequenceAnglesUnits=deg  RotationMatrix=[1 0 0; 0 1 0; 0 0 1]
  motor-position5 : sm_lib/Frames and Transforms/Rigid Transform  TranslationMethod=Cylindrical  TranslationStandardOffset=0  TranslationLengthUnit=m  TranslationStandardAxis=+Z  TranslationCartesianOffset=[0.14 0.14 0.03]  TranslationROffset=arm_length  TranslationROffsetUnits=m  TranslationZOffset=0.03  TranslationZOffsetUnits=m  TranslationThetaOffset=-150  TranslationThetaOffsetUnits=deg  RotationMethod=StandardAxis  RotationAngleUnits=deg  RotationStandardAxis=+Y  RotationAngle=0.0  RotationArbitraryAxis=[0 0 1]  FollAlignAxisA=+X  BaseAlignAxisA=+Y  FollAlignAxisB=+Y  BaseAlignAxisB=+Z  RotationSequenceAxes=FollowerAxes  RotationSequence=XYX  RotationSequenceAngles=[0 0 0]  RotationSequenceAnglesUnits=deg  RotationMatrix=[1 0 0; 0 1 0; 0 0 1]
  motor_black : Subsystem
  motor_cyano : Subsystem
  motor_green : Subsystem
  motor_pink : Subsystem
  motor_red : Subsystem
  motor_yellow : Subsystem
  to_V{,1..5} (6 alike) : Gain  Gain=batVolt/1024
  body_frame : PMIOPort  Side=Left
  motor_velocity : Outport  VectorParamsAs1DForOutWhenUnconnected=off
  Trust_sum : Outport  Port=2  VectorParamsAs1DForOutWhenUnconnected=off
  wires:
  1 - green/1 -> to_V/1
  push right [N]/1 -> motor_green/3(disturb_trust)
  motor_green/2(trust) -> Sum3/1
  motor_red/2(trust) -> Sum3/2
  CV/1 -> motor_green/2(CV_CCV)
  motor-limit1/1 -> motor_green/1(volt)
  CCV/1 -> motor_red/2(CV_CCV)
  Mux/1 -> motor_velocity/1
  Sum3/1 -> Trust_sum/1
  2 - red/1 -> to_V1/1
  motor-limit/1 -> motor_red/1(volt)
  4 yellow/1 -> to_V3/1
  motor-limit2/1 -> motor_yellow/1(volt)
  5 - black/1 -> to_V4/1
  motor-limit3/1 -> motor_black/1(volt)
  CCV1/1 -> motor_black/2(CV_CCV)
  CV1/1 -> motor_yellow/2(CV_CCV)
  motor_yellow/2(trust) -> Sum3/4
  motor_pink/2(trust) -> Sum3/6
  6 - light red/1 -> to_V5/1
  motor-limit4/1 -> motor_pink/1(volt)
  CCV2/1 -> motor_pink/2(CV_CCV)
  3 - light blue/1 -> to_V2/1
  motor-limit5/1 -> motor_cyano/1(volt)
  CCV3/1 -> motor_cyano/2(CV_CCV)
  motor_cyano/2(trust) -> Sum3/3
  motor_green/3(omega) -> Mux/1
  motor_red/3(omega) -> Mux/2
  motor_cyano/3(omega) -> Mux/3
  motor_yellow/3(omega) -> Mux/4
  motor_black/4(omega) -> Mux/5
  motor_pink/3(omega) -> Mux/6
  to_V/1 -> extern voltage/1, motor-limit1/1
  to_V1/1 -> motor-limit/1
  to_V2/1 -> motor-limit5/1
  to_V3/1 -> motor-limit2/1
  to_V4/1 -> motor-limit3/1
  to_V5/1 -> motor-limit4/1
  motor_black/3(trust) -> Sum3/5
  connections:
  motor-position5/LConn1 -- motor-position3/LConn1 -- motor-position4/LConn1 -- motor-position2/LConn1 -- Hex Body/RConn1 -- body_frame/RConn1 -- motor-position/LConn1 -- motor-position1/LConn1
  motor-position1/RConn1 -- motor_green/LConn1
  motor_red/LConn1 -- motor-position/RConn1
  motor_yellow/LConn1 -- motor-position2/RConn1
  motor_black/LConn1 -- motor-position3/RConn1
  motor_pink/LConn1 -- motor-position4/RConn1
  motor_cyano/LConn1 -- motor-position5/RConn1

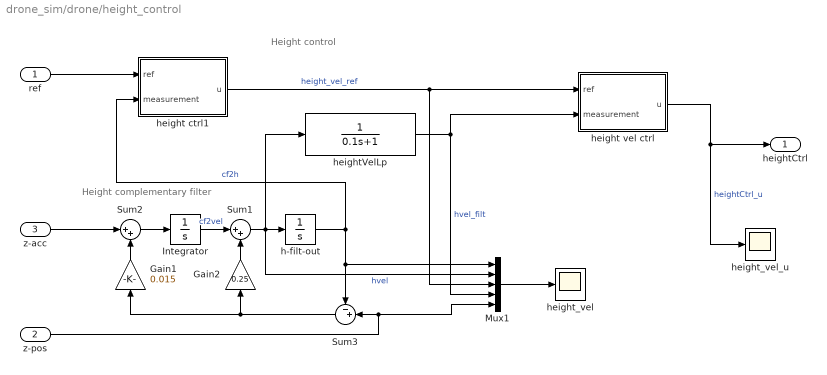
== system drone_sim/drone/height_control ==
  note: Height complementary filter
  note: Height control
  ref : Inport
  z-pos : Inport  Port=2
  z-acc : Inport  Port=3
  Gain1 : Gain  Gain=0.015
  Gain2 : Gain  Gain=0.25
  Integrator : Integrator
  Mux1 : Mux  Inputs=5
  Sum1 : Sum  Inputs=|++
  Sum2 : Sum  Inputs=|++
  Sum3 : Sum  Inputs=-+|
  h-filt-out : Integrator
  height ctrl1 : Subsystem
  height vel ctrl : Subsystem
  heightVelLp : TransferFcn  Denominator=[0.1 1]
  height_vel : Scope
  height_vel_u : Scope
  heightCtrl : Outport
  wires:
  Sum3/1 -> Gain1/1, Gain2/1
  z-pos/1 -> Mux1/5, Sum3/2
  Gain1/1 -> Sum2/2
  height vel ctrl/1(u) -> heightCtrl/1, height_vel_u/1  "heightCtrl_u"
  Sum2/1 -> Integrator/1
  z-acc/1 -> Sum2/1
  Sum1/1 -> heightVelLp/1, Mux1/2, h-filt-out/1  "hvel"
  heightVelLp/1 -> Mux1/4, height vel ctrl/2(measurement)  "hvel_filt"
  Mux1/1 -> height_vel/1
  height ctrl1/1(u) -> Mux1/3, height vel ctrl/1(ref)  "height_vel_ref"
  h-filt-out/1 -> Mux1/1, Sum3/1, height ctrl1/2(measurement)  "cf2h"
  Gain2/1 -> Sum1/2
  Integrator/1 -> Sum1/1  "cf2vel"
  ref/1 -> height ctrl1/1(ref)

== system drone_sim/drone/pitch ctrl ==
  ref : Inport
  measurement : Inport  Port=2
  Gain : Gain  Gain=pakp
  Gain1 : Gain  Commented=on  Gain=1/pati
  Integrator : Integrator  Commented=on  InitialCondition=hoverVoltage  LimitOutput=on  UpperSaturationLimit=batVolt  LowerSaturationLimit=-batVolt
  Sum : Sum  Inputs=|+-
  Sum1 : Sum  Inputs=|++
  Transfer Fcn : TransferFcn  Numerator=[patd 1]  Denominator=[paal*patd 1]
  u : Outport  VectorParamsAs1DForOutWhenUnconnected=off
  wires:
  Gain1/1 -> Integrator/1
  Gain/1 -> Sum1/2, Gain1/1
  Integrator/1 -> Sum1/1
  Sum1/1 -> u/1
  Sum/1 -> Gain/1
  Transfer Fcn/1 -> Sum/2
  measurement/1 -> Transfer Fcn/1
  ref/1 -> Sum/1

== system drone_sim/drone/pitch vel ctrl ==
  ref : Inport
  measurement : Inport  Port=2
  Gain : Gain  Gain=pvkp
  Gain1 : Gain  Commented=on  Gain=pv_iuse/pvti
  Integrator : Integrator  Commented=on  InitialCondition=hoverVoltage  LimitOutput=on  UpperSaturationLimit=500  LowerSaturationLimit=-500
  Sum : Sum  Inputs=|+-
  Sum1 : Sum  Inputs=|++
  Transfer Fcn : TransferFcn  Numerator=[pvtd 1]  Denominator=[pval*pvtd 1]
  u : Outport  VectorParamsAs1DForOutWhenUnconnected=off
  wires:
  ref/1 -> Sum/1
  measurement/1 -> Transfer Fcn/1
  Transfer Fcn/1 -> Sum/2
  Sum/1 -> Gain/1
  Integrator/1 -> Sum1/1
  Gain/1 -> Gain1/1, Sum1/2
  Gain1/1 -> Integrator/1
  Sum1/1 -> u/1

== system drone_sim/drone/roll ctrl ==
  ref : Inport
  measurement : Inport  Port=2
  Gain : Gain  Gain=rakp
  Gain1 : Gain  Commented=on  Gain=1/rati
  Integrator : Integrator  Commented=on  InitialCondition=hoverVoltage  LimitOutput=on  UpperSaturationLimit=batVolt  LowerSaturationLimit=-batVolt
  Sum : Sum  Inputs=|+-
  Sum1 : Sum  Inputs=|++
  Transfer Fcn : TransferFcn  Numerator=[ratd 1]  Denominator=[raal*ratd 1]
  u : Outport  VectorParamsAs1DForOutWhenUnconnected=off
  wires:
  ref/1 -> Sum/1
  measurement/1 -> Transfer Fcn/1
  Transfer Fcn/1 -> Sum/2
  Sum/1 -> Gain/1
  Sum1/1 -> u/1
  Integrator/1 -> Sum1/1
  Gain/1 -> Gain1/1, Sum1/2
  Gain1/1 -> Integrator/1

== system drone_sim/drone/roll vel ctrl ==
  ref : Inport
  measurement : Inport  Port=2
  Gain : Gain  Gain=rkp
  Gain1 : Gain  Commented=on  Gain=1/rti
  Integrator : Integrator  Commented=on  InitialCondition=hoverVoltage  LimitOutput=on  UpperSaturationLimit=batVolt  LowerSaturationLimit=-batVolt
  Sum : Sum  Inputs=|+-
  Sum1 : Sum  Inputs=|++
  Transfer Fcn : TransferFcn  Numerator=[rtd 1]  Denominator=[ral*rtd 1]
  Transfer Fcn1 : TransferFcn  Commented=through  Denominator=[0.02 1]
  u : Outport  VectorParamsAs1DForOutWhenUnconnected=off
  wires:
  Gain1/1 -> Integrator/1
  Gain/1 -> Sum1/2, Gain1/1
  Integrator/1 -> Sum1/1
  Sum/1 -> Gain/1
  Transfer Fcn/1 -> Sum/2
  measurement/1 -> Transfer Fcn/1
  ref/1 -> Sum/1
  Sum1/1 -> Transfer Fcn1/1
  Transfer Fcn1/1 -> u/1

== system drone_sim/drone/yaw vel ctrl ==
  ref : Inport
  measurement : Inport  Port=2
  Gain : Gain  Gain=yawvkp
  Gain1 : Gain  Gain=yawvtiUse/yawvti
  Integrator : Integrator  LimitOutput=on  UpperSaturationLimit=500  LowerSaturationLimit=-500  IgnoreLimit=on
  Sum : Sum  Inputs=|+-
  Sum1 : Sum  Inputs=|++
  Transfer Fcn : TransferFcn  Numerator=[yawvtd 1]  Denominator=[yawval*yawvtd 1]
  u : Outport  VectorParamsAs1DForOutWhenUnconnected=off
  wires:
  Gain1/1 -> Integrator/1
  Gain/1 -> Sum1/2, Gain1/1
  Integrator/1 -> Sum1/1
  Sum/1 -> Gain/1
  measurement/1 -> Transfer Fcn/1  "m"
  ref/1 -> Sum/1
  Sum1/1 -> u/1  "u"
  Transfer Fcn/1 -> Sum/2  "mhat"

== system drone_sim/drone/drone_hardware/Hex Body ==
  arm2 : sm_lib/Frames and Transforms/Rigid Transform  TranslationMethod=None  TranslationStandardOffset=0  TranslationLengthUnit=m  TranslationStandardAxis=+Z  TranslationCartesianOffset=[0 -0.2 0.03]  TranslationROffset=0  TranslationROffsetUnits=m  TranslationZOffset=0  TranslationZOffsetUnits=m  TranslationThetaOffset=0  TranslationThetaOffsetUnits=deg  RotationMethod=StandardAxis  RotationAngleUnits=deg  RotationStandardAxis=+Z  RotationAngle=60  RotationArbitraryAxis=[0 0 1]  FollAlignAxisA=+X  BaseAlignAxisA=+Y  FollAlignAxisB=+Y  BaseAlignAxisB=+Z  RotationSequenceAxes=FollowerAxes  RotationSequence=XYX  RotationSequenceAngles=[0 0 0]  RotationSequenceAnglesUnits=deg  RotationMatrix=[1 0 0; 0 1 0; 0 0 1]
  arm3 : sm_lib/Frames and Transforms/Rigid Transform  TranslationMethod=None  TranslationStandardOffset=0  TranslationLengthUnit=m  TranslationStandardAxis=+Z  TranslationCartesianOffset=[0 -0.2 0.03]  TranslationROffset=0  TranslationROffsetUnits=m  TranslationZOffset=0  TranslationZOffsetUnits=m  TranslationThetaOffset=0  TranslationThetaOffsetUnits=deg  RotationMethod=StandardAxis  RotationAngleUnits=deg  RotationStandardAxis=+Z  RotationAngle=120  RotationArbitraryAxis=[0 0 1]  FollAlignAxisA=+X  BaseAlignAxisA=+Y  FollAlignAxisB=+Y  BaseAlignAxisB=+Z  RotationSequenceAxes=FollowerAxes  RotationSequence=XYX  RotationSequenceAngles=[0 0 0]  RotationSequenceAnglesUnits=deg  RotationMatrix=[1 0 0; 0 1 0; 0 0 1]
  battery : sm_lib/Body Elements/Brick Solid  GraphicAmbientColor=[0.15 0.15 0.15 1.0]  BasedOnType=Mass  BrickDimensions=[0.07 0.15 0.03]  BrickDimensionUnits=m  CenterOfMass=[0 0 0]  CenterOfMassUnits=m  GraphicDiffuseColor=[0.5 0.5 0.5]  Density=1000  DensityUnits=kg/(m^3)  DoExposeReferenceFrame=on  GraphicEmissiveColor=[0.0 0.0 0.0 1.0]  ExportEntireGeometry=off  SerializedFrames=<Frames/>  MarkerShape=Sphere  MarkerSize=10  GraphicType=FromGeometry  InertiaType=CalculateFromGeometry  Mass=batteryMass  MassUnits=kg  MomentsOfInertia=[1 1 1]  MomentsOfInertiaUnits=kg*m^2  GraphicOpacity=1.0  ProductsOfInertia=[0 0 0]  ProductsOfInertiaUnits=kg*m^2  GraphicShininess=75  GraphicSpecularColor=[0.5 0.5 0.5 1.0]  GraphicVisPropType=SimpleVisualProperties
  battery_pos : sm_lib/Frames and Transforms/Rigid Transform  TranslationMethod=Cartesian  TranslationStandardOffset=0  TranslationLengthUnit=m  TranslationStandardAxis=+Z  TranslationCartesianOffset=[0 0 batteryDistanceFromCOG]  TranslationROffset=0  TranslationROffsetUnits=m  TranslationZOffset=0  TranslationZOffsetUnits=m  TranslationThetaOffset=0  TranslationThetaOffsetUnits=deg  RotationMethod=None  RotationAngleUnits=deg  RotationStandardAxis=+Z  RotationAngle=60  RotationArbitraryAxis=[0 0 1]  FollAlignAxisA=+X  BaseAlignAxisA=+Y  FollAlignAxisB=+Y  BaseAlignAxisB=+Z  RotationSequenceAxes=FollowerAxes  RotationSequence=XYX  RotationSequenceAngles=[0 0 0]  RotationSequenceAnglesUnits=deg  RotationMatrix=[1 0 0; 0 1 0; 0 0 1]
  body arm : sm_lib/Body Elements/Brick Solid  GraphicAmbientColor=[0.15 0.15 0.15 1.0]  BasedOnType=Mass  BrickDimensions=[0.04 arm_length*2 0.03]  BrickDimensionUnits=m  CenterOfMass=[0 0 0]  CenterOfMassUnits=m  GraphicDiffuseColor=[0.5 0.5 0.5]  Density=1000  DensityUnits=kg/(m^3)  DoExposeReferenceFrame=on  GraphicEmissiveColor=[0.0 0.0 0.0 1.0]  ExportEntireGeometry=off  SerializedFrames=<Frames/>  MarkerShape=Sphere  MarkerSize=10  GraphicType=FromGeometry  InertiaType=CalculateFromGeometry  Mass=bodyMass/3  MassUnits=kg  MomentsOfInertia=[1 1 1]  MomentsOfInertiaUnits=kg*m^2  GraphicOpacity=1.0  ProductsOfInertia=[0 0 0]  ProductsOfInertiaUnits=kg*m^2  GraphicShininess=75  GraphicSpecularColor=[0.5 0.5 0.5 1.0]  GraphicVisPropType=SimpleVisualProperties
  body1 : sm_lib/Body Elements/Brick Solid  GraphicAmbientColor=[0.15 0.15 0.15 1.0]  BasedOnType=Mass  BrickDimensions=[0.04 arm_length*2 0.03]  BrickDimensionUnits=m  CenterOfMass=[0 0 0]  CenterOfMassUnits=m  GraphicDiffuseColor=[0.5 0.5 0.5]  Density=1000  DensityUnits=kg/(m^3)  DoExposeReferenceFrame=on  GraphicEmissiveColor=[0.0 0.0 0.0 1.0]  ExportEntireGeometry=off  SerializedFrames=<Frames/>  MarkerShape=Sphere  MarkerSize=10  GraphicType=FromGeometry  InertiaType=CalculateFromGeometry  Mass=bodyMass/3  MassUnits=kg  MomentsOfInertia=[1 1 1]  MomentsOfInertiaUnits=kg*m^2  GraphicOpacity=1.0  ProductsOfInertia=[0 0 0]  ProductsOfInertiaUnits=kg*m^2  GraphicShininess=75  GraphicSpecularColor=[0.5 0.5 0.5 1.0]  GraphicVisPropType=SimpleVisualProperties
  body2 : sm_lib/Body Elements/Brick Solid  GraphicAmbientColor=[0.15 0.15 0.15 1.0]  BasedOnType=Mass  BrickDimensions=[0.04 arm_length*2 0.03]  BrickDimensionUnits=m  CenterOfMass=[0 0 0]  CenterOfMassUnits=m  GraphicDiffuseColor=[0.5 0.5 0.5]  Density=1000  DensityUnits=kg/(m^3)  DoExposeReferenceFrame=on  GraphicEmissiveColor=[0.0 0.0 0.0 1.0]  ExportEntireGeometry=off  SerializedFrames=<Frames/>  MarkerShape=Sphere  MarkerSize=10  GraphicType=FromGeometry  InertiaType=CalculateFromGeometry  Mass=bodyMass/3  MassUnits=kg  MomentsOfInertia=[1 1 1]  MomentsOfInertiaUnits=kg*m^2  GraphicOpacity=1.0  ProductsOfInertia=[0 0 0]  ProductsOfInertiaUnits=kg*m^2  GraphicShininess=75  GraphicSpecularColor=[0.5 0.5 0.5 1.0]  GraphicVisPropType=SimpleVisualProperties
  Conn2 : PMIOPort  Side=Right
  connections:
  arm2/LConn1 -- arm3/LConn1 -- Conn2/RConn1 -- battery_pos/LConn1 -- body arm/RConn1
  body2/RConn1 -- arm3/RConn1
  body1/RConn1 -- arm2/RConn1
  battery/RConn1 -- battery_pos/RConn1
